simulink model "Noa_Nofusion_backup"  (R2020b)
settings: Solver=FixedStepDiscrete  StartTime=0.0  StopTime=Inf  FixedStep=0.02  RelTol=1e-3
PostLoadFcn:
  | if any(exist('dsrtsu_mdlpostloadfcn', 'file') ~= 0), dsrtsu_mdlpostloadfcn('Execute', bdroot); end
InitFcn:
  | , if any(exist('rtifpga_mdlclblib', 'file') ~= 0), rtifpga_mdlclblib('Init', bdroot); end,
  | , if any(exist('dsmpb_private', 'file') ~= 0), dsmpb_private('dsmpb_mdlclblib', 'Init', bdroot); end,
undefined symbols (not defined in the file): ACC_TimeGap_DecSetSwt, ACC_TimeGap_IncSetSwt, AccelPedalPosn, AccelPedalPosnVldty, AccelPedlPosnDiagc, AccPedalOverride, ACU_ShiftInProgress, ADAS_Posn_CurLane, AESSwtReq, ALC_SwtReq, BrkPedalSts, CC_ACC_CANCEL_OFFSwt, CC_ACC_CRUISE_OFFSwt, CC_ACC_DecSetSpd_SetSwt, CC_ACC_IncSetSpd_ResuSwt, CC_ACCSwtErr, CharSpd_ms, CSA_NODE, CURRENT_GEAR, CurrentGearValid, DiscIntNeverNeededParam, DrvDoorSts, DrvSBR, DrvTrqReqOvld, ECMACCInterface, ECMRespACC, ELKSwtReq, EngLimpHomeSts, EngSpd, EngState, EngState_PHEV, EngTrqMaxActSpd, EngTrqMinAct, EPS_DrvInpTrqVal_HighReslolution, EPS_FailSts, EPS_LKATorqOvrlDlvd, EPS_LKATorqOvrlDlvdVld, EPS_LKATrqOvlDlvdSts, EPS_SteerMod, EPS_TrqSnsrSts, EQ4_APPINFO, EQ4_LA_ELEM, EQ4_LA_HDR, EQ4_LAP_ELEM, EQ4_LAP_HDR, EQ4_LH_ELEM, EQ4_LH_HDR, EQ4_LRE_ELEM, EQ4_LRE_HDR, ESS_PedSwtReq, ESS_VehSwtReq, FFogLmpSts_F_Pbox, FLWheelDriveDirection, FLWheelSpd, FrntWiprSwtSts, FrntWshrSwtSts, FRWheelDriveDirection, FRWheelSpd, HazardLmpSwtSts, HCU_AccelPedalPosn_Diag ... (+152)
libraries: simulink x117, dsmpblib x30
(part 11 of 11)

== matlab function Noa_Nofusion_backup/Subsystem4/LALine ==
  data: LA_Count input; L1Conf output uint8 size=1; L1C0 output single size=1; L1C1 output single size=1; L1C2 output single size=1; L1C3 output single size=1; L1DxMin output single size=1; L1DxMax output single size=1; L1A0 input single size=1; L1A1 input single size=1; L1A2 input single size=1; L1A3 input single size=1; L1RaMin input single size=1; L1RaMax input single size=1; L1Avail input uint8 size=1; L1LineType input uint8 size=1; L1DLType input uint8 size=1; L1SideType input uint8 size=1; L1Wid input single size=1; L1Confidence input; L2A0 input single size=1; L2A1 input single size=1; L2A2 input single size=1; L2A3 input single size=1; L2RaMin input single size=1; L2RaMax input single size=1; L2Avail input uint8 size=1; L2LineType input uint8 size=1; L2DLType input uint8 size=1; L2SideType input uint8 size=1; L2Wid input single size=1; L2Confidence input; L3A0 input single size=1; L3A1 input single size=1; L3A2 input single size=1; L3A3 input single size=1; L3RaMin input single size=1; L3RaMax input single size=1; L3Avail input uint8 size=1; L3LineType input uint8 size=1; L3DLType input uint8 size=1; L3SideType input uint8 size=1; L3Wid input single size=1; L3Confidence input; L4A0 input single size=1; L4A1 input single size=1; L4A2 input single size=1; L4A3 input single size=1; L4RaMin input single size=1; L4RaMax input single size=1; L4Avail input uint8 size=1; L4LineType input uint8 size=1; L4DLType input uint8 size=1; L4SideType input uint8 size=1; L4Wid input single size=1; L1Type output uint8 size=1; L1DLM output uint8 size=1; L1Width output single size=1; L1Reliable output; L2Conf output uint8 size=1; L2C0 output single size=1; L2C1 output single size=1; L2C2 output single size=1; L2C3 output single size=1; L2DxMin output single size=1; L2DxMax output single size=1; L2Type output uint8 size=1; L2DLM output uint8 size=1; L2Width output single size=1; L2Reliable output; L3Conf output uint8 size=1; L3C0 output single size=1; L3C1 output single size=1; L3C2 output single size=1; L3C3 output single size=1; L3DxMin output single size=1; L3DxMax output single size=1; L3Type output uint8 size=1; L3DLM output uint8 size=1; L3Width output single size=1; L3Reliable output; L4Conf output uint8 size=1; L4C0 output single size=1; L4C1 output single size=1; L4C2 output single size=1; L4C3 output single size=1; L4DxMin output single size=1; L4DxMax output single size=1; L4Type output uint8 size=1; L4DLM output uint8 size=1; L4Width output single size=1; L4Confidence input; L4Reliable output
function [L1Conf,L1C0,L1C1,L1C2,L1C3,L1DxMin,L1DxMax,L1Type,L1DLM,L1Width,L1Reliable,...
    L2Conf,L2C0,L2C1,L2C2,L2C3,L2DxMin,L2DxMax,L2Type,L2DLM,L2Width,L2Reliable,...
    L3Conf,L3C0,L3C1,L3C2,L3C3,L3DxMin,L3DxMax,L3Type,L3DLM,L3Width,L3Reliable,...
    L4Conf,L4C0,L4C1,L4C2,L4C3,L4DxMin,L4DxMax,L4Type,L4DLM,L4Width,L4Reliable]...
    = LA(LA_Count,L1A0,L1A1,L1A2,L1A3,L1RaMin,L1RaMax,L1Avail,L1LineType,L1DLType,L1SideType,L1Wid,L1Confidence,...
    L2A0,L2A1,L2A2,L2A3,L2RaMin,L2RaMax,L2Avail,L2LineType,L2DLType,L2SideType,L2Wid,L2Confidence,...
    L3A0,L3A1,L3A2,L3A3,L3RaMin,L3RaMax,L3Avail,L3LineType,L3DLType,L3SideType,L3Wid,L3Confidence,...
    L4A0,L4A1,L4A2,L4A3,L4RaMin,L4RaMax,L4Avail,L4LineType,L4DLType,L4SideType,L4Wid,L4Confidence)

L1Conf = uint8(0);
L1C0 = single(0);
L1C1 = single(0);
L1C2 = single(0);
L1C3 = single(0);
L1DxMin = single(0);
L1DxMax = single(0);
L1Type = uint8(0);
L1DLM = uint8(0);
L1Width = single(0);
L1Reliable = single(0);

L2Conf = uint8(0);
L2C0 = single(0);
L2C1 = single(0);
L2C2 = single(0);
L2C3 = single(0);
L2DxMin = single(0);
L2DxMax = single(0);
L2Type = uint8(0);
L2DLM = uint8(0);
L2Width = single(0);
L2Reliable = single(0);

L3Conf = uint8(0);
L3C0 = single(0);
L3C1 = single(0);
L3C2 = single(0);
L3C3 = single(0);
L3DxMin = single(0);
L3DxMax = single(0);
L3Type = uint8(0);
L3DLM = uint8(0);
L3Width = single(0);
L3Reliable = single(0);

L4Conf = uint8(0);
L4C0 = single(0);
L4C1 = single(0);
L4C2 = single(0);
L4C3 = single(0);
L4DxMin = single(0);
L4DxMax = single(0);
L4Type = uint8(0);
L4DLM = uint8(0);
L4Width = single(0);
L4Reliable = single(0);
%%  临车道车道线预处理
if LA_Count >= 1                                     %临车道车道线数量
    if L1SideType==1                                 %左左车道线
        L1Conf = L1Avail;
        L1C0 = L1A0;
        L1C1 = L1A1;
        L1C2 = L1A2;
        L1C3 = L1A3;
        L1DxMin = L1RaMin;
        L1DxMax = L1RaMax;
        L1Type = L1LineType;
        L1DLM = L1DLType;
        L1Width = L1Wid;
        L1Reliable = L1Confidence;
    elseif L1SideType==2                             %左车道右侧车道线
        L2Conf = L1Avail;
        L2C0 = L1A0;
        L2C1 = L1A1;
        L2C2 = L1A2;
        L2C3 = L1A3;
        L2DxMin = L1RaMin;
        L2DxMax = L1RaMax;
        L2Type = L1LineType;
        L2DLM = L1DLType;
        L2Width = L1Wid;
        L2Reliable = L1Confidence;
    elseif L1SideType==3                             %右车道左侧车道线
        L3Conf = L1Avail;
        L3C0 = L1A0;
        L3C1 = L1A1;
        L3C2 = L1A2;
        L3C3 = L1A3;
        L3DxMin = L1RaMin;
        L3DxMax = L1RaMax;
        L3Type = L1LineType;
        L3DLM = L1DLType;
        L3Width = L1Wid;
        L3Reliable = L1Confidence;
    elseif L1SideType==4                             %右右车道线
        L4Conf = L1Avail;
        L4C0 = L1A0;
        L4C1 = L1A1;
        L4C2 = L1A2;
        L4C3 = L1A3;
        L4DxMin = L1RaMin;
        L4DxMax = L1RaMax;
        L4Type = L1LineType;
        L4DLM = L1DLType;
        L4Width = L1Wid;
        L4Reliable = L1Confidence;
    end
    if LA_Count >= 2
        if L2SideType==1
            L1Conf = L2Avail;
            L1C0 = L2A0;
            L1C1 = L2A1;
            L1C2 = L2A2;
            L1C3 = L2A3;
            L1DxMin = L2RaMin;
            L1DxMax = L2RaMax;
            L1Type = L2LineType;
            L1DLM = L2DLType;
            L1Width = L2Wid;
            L1Reliable = L2Confidence;
        elseif L2SideType==2
            L2Conf = L2Avail;
            L2C0 = L2A0;
            L2C1 = L2A1;
            L2C2 = L2A2;
            L2C3 = L2A3;
            L2DxMin = L2RaMin;
            L2DxMax = L2RaMax;
            L2Type = L2LineType;
            L2DLM = L2DLType;
            L2Width = L2Wid;
            L2Reliable = L2Confidence;
        elseif L2SideType==3
            L3Conf = L2Avail;
            L3C0 = L2A0;
            L3C1 = L2A1;
            L3C2 = L2A2;
            L3C3 = L2A3;
            L3DxMin = L2RaMin;
            L3DxMax = L2RaMax;
            L3Type = L2LineType;
            L3DLM = L2DLType;
            L3Width = L2Wid;
            L3Reliable = L2Confidence;
        elseif L2SideType==4
            L4Conf = L2Avail;
            L4C0 = L2A0;
            L4C1 = L2A1;
            L4C2 = L2A2;
            L4C3 = L2A3;
            L4DxMin = L2RaMin;
            L4DxMax = L2RaMax;
            L4Type = L2LineType;
            L4DLM = L2DLType;
            L4Width = L2Wid;
            L4Reliable = L2Confidence;
        end
        if LA_Count >= 3
            if L3SideType==1
                L1Conf = L3Avail;
                L1C0 = L3A0;
                L1C1 = L3A1;
                L1C2 = L3A2;
                L1C3 = L3A3;
                L1DxMin = L3RaMin;
                L1DxMax = L3RaMax;
                L1Type = L3LineType;
                L1DLM = L3DLType;
                L1Width = L3Wid;
                L1Reliable = L3Confidence;
            elseif L3SideType==2
                L2Conf = L3Avail;
                L2C0 = L3A0;
                L2C1 = L3A1;
                L2C2 = L3A2;
                L2C3 = L3A3;
                L2DxMin = L3RaMin;
                L2DxMax = L3RaMax;
                L2Type = L3LineType;
                L2DLM = L3DLType;
                L2Width = L3Wid;
                L2Reliable = L3Confidence;
            elseif L3SideType==3
                L3Conf = L3Avail;
                L3C0 = L3A0;
                L3C1 = L3A1;
                L3C2 = L3A2;
                L3C3 = L3A3;
                L3DxMin = L3RaMin;
                L3DxMax = L3RaMax;
                L3Type = L3LineType;
                L3DLM = L3DLType;
                L3Width = L3Wid;
                L3Reliable = L3Confidence;
            elseif L3SideType==4
                L4Conf = L3Avail;
                L4C0 = L3A0;
                L4C1 = L3A1;
                L4C2 = L3A2;
                L4C3 = L3A3;
                L4DxMin = L3RaMin;
                L4DxMax = L3RaMax;
                L4Type = L3LineType;
                L4DLM = L3DLType;
                L4Width = L3Wid;
                L4Reliable = L3Confidence;
            end
            if LA_Count >= 4
                if L4SideType==1
                    L1Conf = L4Avail;
                    L1C0 = L4A0;
                    L1C1 = L4A1;
                    L1C2 = L4A2;
                    L1C3 = L4A3;
                    L1DxMin = L4RaMin;
                    L1DxMax = L4RaMax;
                    L1Type = L4LineType;
                    L1DLM = L4DLType;
                    L1Width = L4Wid;
                    L1Reliable = L4Confidence;
                elseif L4SideType==2
                    L2Conf = L4Avail;
                    L2C0 = L4A0;
                    L2C1 = L4A1;
                    L2C2 = L4A2;
                    L2C3 = L4A3;
                    L2DxMin = L4RaMin;
                    L2DxMax = L4RaMax;
                    L2Type = L4LineType;
                    L2DLM = L4DLType;
                    L2Width = L4Wid;
                    L2Reliable = L4Confidence;
                elseif L4SideType==3
                    L3Conf = L4Avail;
                    L3C0 = L4A0;
                    L3C1 = L4A1;
                    L3C2 = L4A2;
                    L3C3 = L4A3;
                    L3DxMin = L4RaMin;
                    L3DxMax = L4RaMax;
                    L3Type = L4LineType;
                    L3DLM = L4DLType;
                    L3Width = L4Wid;
                    L3Reliable = L4Confidence;
                elseif L4SideType==4
                    L4Conf = L4Avail;
                    L4C0 = L4A0;
                    L4C1 = L4A1;
                    L4C2 = L4A2;
                    L4C3 = L4A3;
                    L4DxMin = L4RaMin;
                    L4DxMax = L4RaMax;
                    L4Type = L4LineType;
                    L4DLM = L4DLType;
                    L4Width = L4Wid;
                    L4Reliable = L4Confidence;
                end
            end
        end
    end
end

== stateflow chart Noa_Nofusion_backup/Common/Subsystem7/DS/DriverSts_StateMachine ==
  state DriverSts [group]
    0x0:DriverUnbeliv
    0x1:DriverGood
    0x2:DriverLowDistractn
    0x3:DriverMidDistractn
    0x4:DriverHi1Distractn
    0x5:DriverHi2Distractn
    0x6:DriverLowDrowsiness
    0x7:DriverMidDrowsiness
    0x8:DriverHi1Drowsiness
    0x9:DriverHi2Drowsiness
  state DistractnSts [group]
    0x0:DMSNoDistractn
    0x1:DMSLowDistractn
    0x2:DMSMidDistractn
    0x3:DMSHi1Distractn
    0x4:DMSHi2Distractn
    0x5:DMSUnbelievDistractn
    DrowsnsSts
    0x0:DMSNoDrowsiness
    0x1:DMSLowDrowsiness
    0x2:DMSMidDrowsiness
    0x3:DMSHi1Drowsiness
    0x4:DMSHi2Drowsiness
    0x5:DMSUnbelievDrowsiness
  state Ini
    entry: DriverSts=DriverUnbeliv;
    DADistractnNoDistractn=0;
    DADrowsnsNoDrowsiness=0;
  state Unbelievable
    entry: DriverSts=DriverUnbeliv;
    DistractnSts=DMSUnbelievDistractn;
    DrowsnsSts=DMSUnbelievDrowsiness;
  state Good
    entry:DriverSts=DriverGood;
    DistractnSts=DMSNoDistractn;
    DrowsnsSts=DMSNoDrowsiness;
  state DDA
    state Distractn [parallel]
      settings: executionOrder=1
      state NoDis
        entry:DistractnSts=DMSNoDistractn;
        DADistractnNoDistractn=1;
        exit:DADistractnNoDistractn=0;
      state ExistDis
        state LowDis
          entry:DistractnSts=DMSLowDistractn;
        state MidDis
          entry:DistractnSts=DMSMidDistractn;
        state Hi1Dis
          entry:DistractnSts=DMSHi1Distractn;
        state Hi2Dis
          entry:DistractnSts=DMSHi2Distractn;
        LowDis -> (junction 143) [order 2] : [DSOther2Hi1Distractn]
        (junction 143) -> (junction 126)
        (default) -> (junction 137)
        (junction 137) -> LowDis [order 1] : [DSGoodUnbeliv2LowDistractn]
        (junction 146) -> LowDis
        (junction 147) -> (junction 146)
        (junction 137) -> (junction 142) [order 2]
        (junction 144) -> (junction 146) [order 1] : [DSMidHi1Hi22LowDistractn]
        (junction 124) -> (junction 147) [order 1] : [DSMidHi1Hi22LowDistractn]
        LowDis -> MidDis [order 1] : [DSLow2MidDistractn]
        MidDis -> LowDis [order 2] : [DSMidHi1Hi22LowDistractn]
        (junction 142) -> MidDis [order 1] : [DSGoodUnbeliv2MidDistractn]
        (junction 144) -> MidDis [order 2]
        (junction 124) -> (junction 144) [order 2]
        (junction 142) -> (junction 138) [order 2]
        Hi2Dis -> (junction 144) : [DSHi1Hi22MidDistractn||......
            | DSMidHi1Hi22LowDistractn]
        (junction 130) -> (junction 124)
        MidDis -> Hi1Dis [order 1] : [DSOther2Hi1Distractn]
        Hi1Dis -> MidDis [order 2] : [DSHi1Hi22MidDistractn]
        Hi1Dis -> Hi2Dis [order 1] : [DSOther2Hi2Distractn]
        (junction 138) -> Hi1Dis
        (junction 126) -> Hi1Dis
        Hi1Dis -> (junction 130) [order 3] : [DSHi1Hi22MidDistractn||......
            | DSMidHi1Hi22LowDistractn]
      (default) -> (junction 122)
      (junction 122) -> NoDis [order 2]
      (junction 122) -> ExistDis [order 1] : [DSGoodUnbeliv2LowDistractn||......
          | DSGoodUnbeliv2MidDistractn||......
          | DSOther2Hi1Distractn]
      NoDis -> ExistDis : [DSGoodUnbeliv2LowDistractn||......
          | DSGoodUnbeliv2MidDistractn||......
          | DSOther2Hi1Distractn]
      ExistDis -> NoDis : [DSMidHi1Hi22NoDistractn]
    state Drowsns [parallel]
      settings: executionOrder=2
      state NoDrow
        entry:DrowsnsSts=DMSNoDrowsiness;
        DADrowsnsNoDrowsiness=1;
        exit:DADrowsnsNoDrowsiness=0;
      state ExistDrow
        state LowDrow
          entry:DrowsnsSts=DMSLowDrowsiness;
        state MidDrow
          entry:DrowsnsSts=DMSMidDrowsiness;
        state Hi1Drow
          entry:DrowsnsSts=DMSHi1Drowsiness;
        state Hi2Drow
          entry:DrowsnsSts=DMSHi2Drowsiness;
        LowDrow -> (junction 58) [order 2] : [DSOther2Hi1Drowsns]
        (junction 58) -> (junction 46)
        (default) -> (junction 36)
        (junction 36) -> LowDrow [order 1] : [DSGoodUnbeliv2LowDrowsns]
        (junction 10) -> LowDrow
        (junction 74) -> (junction 10)
        (junction 36) -> (junction 42) [order 2]
        (junction 11) -> (junction 10) [order 1] : [DSMidHi1Hi22LowDrowsns]
        (junction 61) -> (junction 74) [order 1] : [DSMidHi1Hi22LowDrowsns]
        LowDrow -> MidDrow [order 1] : [DSLow2MidDrowsns]
        MidDrow -> LowDrow [order 2] : [DSMidHi1Hi22LowDrowsns]
        (junction 42) -> MidDrow [order 1] : [DSGoodUnbeliv2MidDrowsns]
        (junction 11) -> MidDrow [order 2]
        (junction 61) -> (junction 11) [order 2]
        (junction 42) -> (junction 59) [order 2]
        Hi2Drow -> (junction 11) : [DSMidHi1Hi22LowDrowsns||......
            | DSHi1Hi22MidDrowsns]
        (junction 39) -> (junction 61)
        MidDrow -> Hi1Drow [order 1] : [DSOther2Hi1Drowsns]
        Hi1Drow -> MidDrow [order 2] : [DSHi1Hi22MidDrowsns]
        Hi1Drow -> Hi2Drow [order 1] : [DSOther2Hi2Drowsns]
        (junction 59) -> Hi1Drow
        (junction 46) -> Hi1Drow
        Hi1Drow -> (junction 39) [order 3] : [DSMidHi1Hi22LowDrowsns||......
            | DSHi1Hi22MidDrowsns]
      (default) -> (junction 72)
      (junction 72) -> NoDrow [order 2]
      (junction 72) -> ExistDrow [order 1] : [DSGoodUnbeliv2LowDrowsns||......
          | DSGoodUnbeliv2MidDrowsns||......
          | DSOther2Hi1Drowsns]
      NoDrow -> ExistDrow : [DSGoodUnbeliv2LowDrowsns||......
          | DSGoodUnbeliv2MidDrowsns||......
          | DSOther2Hi1Drowsns]
      ExistDrow -> NoDrow : [DSMidHi1Hi22NoDrowsns]
    state Arbitrate [parallel]
      settings: executionOrder=3
      Arbitrate -> (junction 20)
      (junction 20) -> (junction 75) [order 1] : [DistractnSts<DrowsnsSts]
      (junction 75) -> (junction 45) [order 1] : [DrowsnsSts==DMSHi2Drowsiness]
          | {DriverSts=DriverHi2Drowsiness;}
      (junction 20) -> (junction 14) [order 2]
      (junction 75) -> (junction 54) [order 2]
      (junction 45) -> (junction 19)
      (junction 14) -> (junction 48) [order 1] : [DistractnSts==DMSHi2Distractn]
          | {DriverSts=DriverHi2Distractn;}
      (junction 54) -> (junction 19) [order 1] : [DrowsnsSts==DMSHi1Drowsiness]
          | {DriverSts=DriverHi1Drowsiness;}
      (junction 14) -> (junction 89) [order 2]
      (junction 48) -> (junction 1)
      (junction 54) -> (junction 4) [order 2]
      (junction 19) -> (junction 5)
      (junction 89) -> (junction 1) [order 1] : [DistractnSts==DMSHi1Distractn]
          | {DriverSts=DriverHi1Distractn;}
      (junction 4) -> (junction 5) [order 1] : [DrowsnsSts==DMSMidDrowsiness]
          | {DriverSts=DriverMidDrowsiness;}
      (junction 89) -> (junction 95) [order 2]
      (junction 1) -> (junction 105)
      (junction 4) -> (junction 97) [order 2] : {DriverSts=DriverLowDrowsiness;}
      (junction 5) -> (junction 102)
      (junction 95) -> (junction 105) [order 1] : [DistractnSts==DMSMidDistractn]
          | {DriverSts=DriverMidDistractn;}
      (junction 105) -> (junction 93)
      (junction 95) -> (junction 99) [order 2] : {DriverSts=DriverLowDistractn;}
      (junction 93) -> (junction 99)
      (junction 97) -> (junction 93)
      (junction 102) -> (junction 97)
      (junction 99) -> Arbitrate
  (default) -> Ini
  Ini -> Unbelievable
  Unbelievable -> Good [order 2] : [DSOther2Good]
  Good -> Unbelievable [order 1] : [DSOther2Unbeliv]
  Unbelievable -> DDA [order 1] : [(DSGoodUnbeliv2LowDistractn||......
      | DSGoodUnbeliv2MidDistractn||......
      | DSOther2Hi1Distractn||......
      | DSGoodUnbeliv2LowDrowsns||......
      | DSGoodUnbeliv2MidDrowsns||......
      | DSOther2Hi1Drowsns)&&......
      | DSUnbeliv2DDAEnable]
  DDA -> Unbelievable [order 1] : [DSOther2Unbeliv]
  DDA -> Good [order 2] : [DSOther2Good||(DADistractnNoDistractn&&DADrowsnsNoDrowsiness)]
  Good -> DDA [order 2] : [DSGoodUnbeliv2LowDistractn||......
      | DSGoodUnbeliv2MidDistractn||......
      | DSOther2Hi1Distractn||......
      | DSGoodUnbeliv2LowDrowsns||......
      | DSGoodUnbeliv2MidDrowsns||......
      | DSOther2Hi1Drowsns]
  data: DSOther2Good input; DSOther2Unbeliv input; DADistractnNoDistractn local uint8; DADrowsnsNoDrowsiness local uint8; DistractnSts output uint8 =uint8(0); DrowsnsSts output uint8 =uint8(0); DMSHi1Distractn local uint8 =uint8(3); DMSHi1Drowsiness local uint8 =uint8(3); DMSHi2Distractn local uint8 =uint8(4); DMSHi2Drowsiness local uint8 =uint8(4); DMSLowDistractn local uint8 =uint8(1); DMSLowDrowsiness local uint8 =uint8(1); DMSMidDistractn local uint8 =uint8(2); DMSMidDrowsiness local uint8 =uint8(2); DMSNoDistractn local uint8 =uint8(0); DMSNoDrowsiness local uint8 =uint8(0); DMSUnbelievDistractn local uint8 =uint8(5); DMSUnbelievDrowsiness local uint8 =uint8(5); DriverGood local uint8 =uint8(1); DriverHi1Distractn local uint8 =uint8(4); DriverHi1Drowsiness local uint8 =uint8(8); DriverHi2Distractn local uint8 =uint8(5); DriverHi2Drowsiness local uint8 =uint8(9); DriverLowDistractn local uint8 =uint8(2); DriverLowDrowsiness local uint8 =uint8(6); DriverMidDistractn local uint8 =uint8(3); DriverMidDrowsiness local uint8 =uint8(7); DriverSts output uint8; DriverUnbeliv local uint8 =uint8(0); DSGoodUnbeliv2LowDistractn input; DSMidHi1Hi22LowDistractn input; DSGoodUnbeliv2MidDistractn input; DSLow2MidDistractn input; DSHi1Hi22MidDistractn input; DSOther2Hi1Distractn input; DSOther2Hi2Distractn input; DSGoodUnbeliv2LowDrowsns input; DSMidHi1Hi22LowDrowsns input; DSGoodUnbeliv2MidDrowsns input; DSLow2MidDrowsns input; DSHi1Hi22MidDrowsns input; DSOther2Hi1Drowsns input; DSOther2Hi2Drowsns input; DSMidHi1Hi22NoDistractn input; DSMidHi1Hi22NoDrowsns input; DSUnbeliv2DDAEnable input

== matlab function Noa_Nofusion_backup/Subsystem2/ACCOSM/HWA_Task100ms1/ACC_DisplayBar ==
  data: TimeGap input; DisplayBar output uint8; DesireDistance input; ACCmode input; TargetRange input; Scale input; TargetExist input; DisplayBarK1 input uint8
function DisplayBar = fcn(TimeGap,DesireDistance,ACCmode,TargetRange,Scale,TargetExist,DisplayBarK1)
%#codegen
DisplayBar = DisplayBarK1;

ScaleDis = Scale*DesireDistance;
upScaleDis = (Scale+single(0.05))*DesireDistance;
lowScaleDis = (Scale-single(0.05))*DesireDistance;

i = TimeGap;

if (ACCmode==0)||(ACCmode==7)
    DisplayBar = uint8(0);
else
    if TargetExist==false
        DisplayBar=uint8(0);
    else
        switch(DisplayBarK1)
            case uint8(0)
                 if TargetRange> ScaleDis(i,3)
                     DisplayBar=uint8(4);
                 else
                     if TargetRange>ScaleDis(i,2)
                         DisplayBar=uint8(3);
                     else
                         if TargetRange>ScaleDis(i,1)
                             DisplayBar=uint8(2);
                         else
                             DisplayBar=uint8(1);
                         end
                     end
                 end
            case uint8(1)
                 if TargetRange> upScaleDis(i,3)
                     DisplayBar=uint8(4);
                 else
                     if TargetRange>upScaleDis(i,2)
                         DisplayBar=uint8(3);
                     else
                         if TargetRange>upScaleDis(i,1)
                             DisplayBar=uint8(2);
                         else
                             DisplayBar=uint8(1);
                         end
                     end
                 end
            case uint8(2)
                 if TargetRange> upScaleDis(i,3)
                     DisplayBar=uint8(4);
                 else
                     if TargetRange>upScaleDis(i,2)
                         DisplayBar=uint8(3);
                     else
                         if TargetRange>lowScaleDis(i,1)
                             DisplayBar=uint8(2);
                         else
                             DisplayBar=uint8(1);
                         end
                     end
                 end   
            case uint8(3)
                 if TargetRange> upScaleDis(i,3)
                     DisplayBar=uint8(4);
                 else
                     if TargetRange>lowScaleDis(i,2)
                         DisplayBar=uint8(3);
                     else
                         if TargetRange>lowScaleDis(i,1)
                             DisplayBar=uint8(2);
                         else
                             DisplayBar=uint8(1);
                         end
                     end
                end
            case uint8(4)
                 if TargetRange> lowScaleDis(i,3)
                     DisplayBar=uint8(4);
                 else
                     if TargetRange>lowScaleDis(i,2)
                         DisplayBar=uint8(3);
                     else
                         if TargetRange>lowScaleDis(i,1)
                             DisplayBar=uint8(2);
                         else
                             DisplayBar=uint8(1);
                         end
                     end
                 end      
        end    
    end
end

== matlab function Noa_Nofusion_backup/Subsystem2/ACCOSM/HWA_Task100ms1/Dyc ==
  data: kapTrajFiltK1 input single size=1; vRef input single size=1; kapTrajFilt output single size=1; kapCourseErr output single; kapTraj input single size=1; alpSideSlipAngle input single size=1; A2 input single size=1; A1 input single size=1; LineValid input boolean size=1; ObjDx input single size=15; ObjDy input single size=15; TarLineValid input boolean; TarLineA2 input single; TarLineA1 input single; TarLineA0 input single size=1; dxC0 output single size=1; aPC0 output single size=1; bPC0 output single size=1; cPC0 output single size=1; aPC1 output single size=1; bPC1 output single size=1; cPC1 output single size=1; ObjDyc output single size=15
function [kapTrajFilt,kapCourseErr,dxC0,aPC0,bPC0,cPC0,aPC1,bPC1,cPC1,ObjDyc] = ...
    DriveCourseCalc(kapTrajFiltK1,vRef,kapTraj,alpSideSlipAngle,...
    A2,A1,LineValid,ObjDx,ObjDy,TarLineValid,TarLineA2,TarLineA1,TarLineA0)

ObjDyc = single(zeros(15,1));

if vRef>8.33
    t_alpSideSlipAngle = -alpSideSlipAngle;
else
    t_alpSideSlipAngle = single(0);
end

temp1 = single(0.1)/(single(0.1) + interpolate(single(24),single(0),single(55),single(0.4),vRef));

kapTrajFilt = kapTrajFiltK1 + temp1*(kapTraj - kapTrajFiltK1);

temp1 = abs(kapTraj*vRef);

if (temp1<0.001)&&(vRef>8.3)
    t_kapTrajwHyst = single(0);
else
    t_kapTrajwHyst = kapTrajFilt;
end

if TarLineValid
    temp = interpolate(single(0.2),single(0.2),single(1.5),single(1),abs(TarLineA0));
    dxC0Min = single(3);
else
    temp = single(1);
    dxC0Min = single(10);
end

dxC0 = max(vRef*temp,dxC0Min);
aPC0 = 0.5*t_kapTrajwHyst*(single(1)+1.5*t_alpSideSlipAngle*t_alpSideSlipAngle);
bPC0 = t_alpSideSlipAngle;
cPC0 = single(0);

temp1 = single(0.1)*abs(t_kapTrajwHyst);
temp2 = min(single(0.00013),single(0.004)/max(vRef,single(10)));
kapCourseErr = max(temp1,temp2);

aPC1 = aPC0;
bPC1 = bPC0;
cPC1 = single(0);

Low = interpolate(single(4),single(1),single(20),single(0),abs(atan(A1)));    % low vehiclespeed lanechange Angle is 4deg~20deg;
High = interpolate(single(4),single(1),single(10),single(0),abs(atan(A1)));   % low vehiclespeed lanechange Angle is 4deg~10deg;
t_vRefFactor = interpolate(single(5),Low,single(25),High,vRef);

t_Factor = single(1)*t_vRefFactor;

if TarLineValid==true
    aPC1 = TarLineA2;
    bPC1 = TarLineA1;
    cPC1 = (aPC0 - aPC1)*dxC0*dxC0 + (bPC0 - bPC1)*dxC0;
else
    if LineValid
        aPC1 = aPC0*(1 - t_Factor) + A2*t_Factor;
        bPC1 = bPC0*(1 - t_Factor) + A1*t_Factor;
        cPC1 = (aPC0 - aPC1)*dxC0*dxC0 + (bPC0 - bPC1)*dxC0;
    end
end

for i=1:15
   if ObjDx(i)>dxC0
      ObjDyc(i) =  ObjDy(i) - (aPC1*ObjDx(i)*ObjDx(i) + bPC1*ObjDx(i) + cPC1);
   else
      ObjDyc(i) =  ObjDy(i) - (aPC0*ObjDx(i)*ObjDx(i) + bPC0*ObjDx(i));
   end
end
end


function out = interpolate(x1,z1,x2,z2,Raw)
if Raw<=x1
    out = z1;
else
    if Raw>=x2
        out = z2;
    else
        out = z1 + (Raw-x1)*(z2-z1)/(x2-x1);
    end
end
end

== matlab function Noa_Nofusion_backup/Subsystem2/ACCOSM/HWA_Task100ms1/DycCutIn ==
  data: ObjValid input boolean size=15; ObjDyc input single size=15; ObjMoveSts input uint8 size=15; ObjDycCutIn output single size=15; ObjMove_b output boolean size=15; ObjCnt input uint8 size=15; ObjDycHist input single size=15; ObjqDycHist input single size=15; dycFiltK1 input single size=15; ObjDycFilt output single size=15
function [ObjDycCutIn,ObjMove_b,ObjDycFilt] = ...
    ObjDycCutInCalc(ObjValid,ObjDyc,ObjMoveSts,ObjCnt,ObjDycHist,ObjqDycHist,dycFiltK1)
 
ObjDycCutIn = single(zeros(15,1));
ObjDycFilt = single(zeros(15,1));
ObjMove_b = false(15,1); 
 
for i=1:15
    if ObjValid(i)
        t_dyc = ObjDyc(i);
        t_dycHist = ObjDycHist(i);
        t_qDycHist = ObjqDycHist(i);
        
        weightDycHist = t_qDycHist*0.1;
        weightDyc = single(1) - weightDycHist;
        
        t_dycASI = weightDycHist*t_dycHist + weightDyc*t_dyc;
        ObjDycCutIn(i) = t_dycASI;
        
        if ObjCnt(i)>2
            ObjDycFilt(i) = 0.028*(t_dycASI - dycFiltK1(i)) + dycFiltK1(i);
        else
            ObjDycFilt(i) = t_dycASI;
        end
        if ObjMoveSts(i)==2
            ObjMove_b(i) = true;
        end
    end
end

== matlab function Noa_Nofusion_backup/Subsystem2/ACCOSM/HWA_Task100ms1/DycHistCalc ==
  data: TrajHistBufferBTrajEnd input boolean; ObjTrajNumber input uint8; ObjDycHist output single; TrajCurrentIndex input uint8; TrajHistBufferBValid input boolean; TrajHistBufferDxv input single; TrajHistBufferDyv input single; ObjValid input boolean; ObjqDycHist output single; dxC0 input; aP0 input; bP0 input; cP0 input; aP1 input; bP1 input; cP1 input
function [ObjDycHist,ObjqDycHist] = DycHistCalc(TrajHistBufferBTrajEnd,ObjTrajNumber,TrajCurrentIndex,...
    TrajHistBufferBValid,TrajHistBufferDxv,TrajHistBufferDyv,ObjValid,dxC0,aP0,bP0,cP0,aP1,bP1,cP1)

t_dxv = single(0);
t_dyv = single(0);
t_dxvK1 = single(0);
t_dyvK1 = single(0);
ObjDycHist = single(zeros(15,1));
ObjqDycHist = single(zeros(15,1));

for iObj=1:15
    t_TrajNumber = ObjTrajNumber(iObj);
    if t_TrajNumber<21
        t_End = false;
        t_Failed = false;
        t_TrajCurrentIndex = TrajCurrentIndex(t_TrajNumber);
        t_TrajEnd = TrajHistBufferBTrajEnd(t_TrajNumber,t_TrajCurrentIndex);
        if (ObjValid(iObj)==true)&&(t_TrajEnd==false)
            for k=1:24
                if t_End==false
                    if t_TrajCurrentIndex<k
                        t_Index = t_TrajCurrentIndex + uint8(25) - k;
                    else
                        t_Index = t_TrajCurrentIndex - k + uint8(1);
                    end
                    if t_Index==1
                        t_IndexK1 = uint8(24);
                    else
                        t_IndexK1 = t_Index - uint8(1);
                    end
                    t_ValidK1 = TrajHistBufferBValid(t_TrajNumber,t_IndexK1);
                    t_TrajEndK1 = TrajHistBufferBTrajEnd(t_TrajNumber,t_IndexK1);
                    t_dxv = TrajHistBufferDxv(t_TrajNumber,t_Index);
                    t_dxvK1 = TrajHistBufferDxv(t_TrajNumber,t_IndexK1);
                    t_dyv = TrajHistBufferDyv(t_TrajNumber,t_Index);
                    t_dyvK1 = TrajHistBufferDyv(t_TrajNumber,t_IndexK1);
                    
                    if (t_TrajEndK1==true)||(t_ValidK1==false)
                        t_End = true;
                        t_Failed = true;
                    end
                    if (t_dxv>=0)&&(t_dxvK1<=0)
                        t_End = true;
                    end
                end
            end
        end
        if (t_End==true)&&(t_Failed==false)
            if (t_dxv==t_dxvK1)
                t_dycHist = t_dyv;
            else
                t_dycHist = t_dyv - t_dxv*(t_dyvK1 - t_dyv)/(t_dxvK1 - t_dxv);
            end
            t_qDycHist = single(1);  
        else
            if (t_End==true)&&(t_Failed==true)&&(t_dxv>0)
                if t_dxv>(dxC0)
                    t_dycHist = t_dyv - (aP1*t_dxv*t_dxv + bP1*t_dxv + cP1); 
                else
                    t_dycHist = t_dyv - (aP0*t_dxv*t_dxv + bP0*t_dxv + cP0); 
                end
               t_qDycHist = max((single(80) - t_dxv)/single(80),single(0));
            else
                t_dycHist = single(0);
                t_qDycHist = single(0);
            end
        end
    else
        t_dycHist = single(0);
        t_qDycHist = single(0);
    end
    ObjDycHist(iObj) = t_dycHist;
    ObjqDycHist(iObj) = t_qDycHist;
end

== matlab function Noa_Nofusion_backup/Subsystem2/ACCOSM/HWA_Task100ms1/LostTargetCalc ==
  data: ObjValid input boolean size=15; ReID output uint8 size=1; ObjDx input single size=15; ObjDy input single size=15; DeltaDx input single size=1; DeltaDy input single size=1; P0IDK1 input uint8 size=1; P0VxK1 input single size=1; P0DxK1 input single size=1; P0DyK1 input single size=1; P0RangeK1 input; P0ArGK1 input; P0DycK1 input single size=1; P0VycK1 input single size=1; P0CutIn_bK1 input boolean size=1; tTargetLostK1 input single size=1; ReRange output single size=1; ReArG output single size=1; ReDx output single size=1; ReDy output single size=1; ReVx output single size=1; ReCutIn_b output boolean size=1; ReDyc output single size=1; ReVyc output single size=1; TargetLost_b output boolean size=1; Covered_b output boolean size=1; tTargetLost output single size=1
function [ReID,ReRange,ReArG,ReDx,ReDy,ReVx,ReCutIn_b,ReDyc,ReVyc,TargetLost_b,Covered_b,tTargetLost]...
    = LostTargetCalc(ObjValid,ObjDx,ObjDy,DeltaDx,DeltaDy,...
    P0IDK1,P0VxK1,P0DxK1,P0DyK1,P0RangeK1,P0ArGK1,P0DycK1,P0VycK1,P0CutIn_bK1,tTargetLostK1)
 
ReID = P0IDK1;
ReRange = single(255);
ReArG = single(0);
ReDx = single(255);
ReDy = single(0);
ReVx = single(0);
ReDyc = single(0);
ReVyc = single(0);
ReCutIn_b = false;
TargetLost_b = false;
tTargetLost = single(0);
Covered_b = false;
 
if (P0IDK1>0)&&(P0IDK1<100)    % k1 Exist Target
    if ObjValid(P0IDK1)==false
        ExistNearObj = false;
        P0DxPred = P0DxK1 + 0.1*P0VxK1;
        P0DyPred = P0DyK1;
        P0RangePred = P0RangeK1 + 0.1*P0VxK1; 
        for i=1:15
            if (ObjValid(i)==true)&&(ObjDx(i)<P0DxPred)
                Covered_b = CoveredCalc(P0DxPred,P0DyPred,ObjDx(i),ObjDy(i),single(2.1),single(-0.1));
                if Covered_b==true
                   break; 
                end
            end
            if (ObjValid(i)==1)&&(abs(ObjDx(i)-P0DxPred)<DeltaDx)&&(abs(ObjDy(i)-P0DyPred)<DeltaDy)
               ExistNearObj = true;
               ReID = uint8(i);
               ReDx = ObjDx(i);
            end
        end
        if (ExistNearObj==false)&&(Covered_b==false)
            TargetLost_b = true;
            tTargetLost = single(0.1);
            ReID = uint8(255);
            ReRange = P0RangePred;
            ReArG = P0ArGK1;
            ReDx = P0DxPred;
            ReDy = P0DyPred;
            ReVx = P0VxK1;
            ReCutIn_b = P0CutIn_bK1;
            ReVyc = P0VycK1;
            ReDyc = P0DycK1 + 0.1*P0VycK1;
        end
    end
else
    if P0IDK1>100   %  k1 Exist Target Re
        ExistNearObj = false;
        P0DxPred = P0DxK1 + 0.1*P0VxK1;
        P0DyPred = P0DyK1;
        P0RangePred = P0RangeK1 + 0.1*P0VxK1; 

        for i=1:15
            if (ObjValid(i)==1)&&(abs(ObjDx(i)-P0DxPred)<DeltaDx)&&(abs(ObjDy(i)-P0DyPred)<DeltaDy)
                ExistNearObj = true;
                ReID = uint8(i);
                ReDx = ObjDx(i);
                TargetLost_b = false;
                tTargetLost = single(0);
            end
        end
        if ExistNearObj==false
            TargetLost_b = true;
            tTargetLost = tTargetLostK1 + single(0.1);
            ReID = uint8(255);
            ReRange = P0RangePred;
            ReArG = P0ArGK1;
            ReDx = P0DxPred;
            ReDy = P0DyPred;
            ReVx = P0VxK1;
            ReCutIn_b = P0CutIn_bK1;
            ReVyc = P0VycK1;
            ReDyc = P0DycK1 + 0.1*P0VycK1;
        end
    end
end
end
 
function t_Covered_b = CoveredCalc(DxPred,DyPred,Dx,Dy,IFVDx,IFVDy)
y = (IFVDy - DyPred)*(Dx - DxPred)/(IFVDx - DxPred) + DyPred ;
Delta = single(0.8) + (Dx - IFVDx)/(DxPred - IFVDx);
if abs(Dy - y)<=Delta
    t_Covered_b = true;
else
    t_Covered_b = false;
end
end
